simulink model "teng4_demo2_UDP_slx2py_sender_DRealTime_okclean"  (R2020a)
settings: Solver=FixedStepDiscrete  StartTime=0.0  StopTime=100  RelTol=1e-3  EnableMultiTasking=on
undefined symbols (not defined in the file or in its folder): Standard_Devices, UDP_Protocol
libraries: sldrtlib x1
Description:
  | Packet Input/Output
  | 
  | The example model "sldrtex_packetio" shows how to transfer data through
  | UDP communication protocol using binary encoding. The model sends data
  | within one computer, from one UDP port to another. You can modify the
  | model to communicate between two computers by splitting this model
  | into its send and receive parts and running the models on two computers.
  | The yellow blocks are used to send the data, the blue blocks
  | are used to receive the data. Then, please enter the host names or
  | IP addresses of the two computers into the appropriate fields
  | in the Board Setup dialog.
  | 
  | How to run this model in Normal Mode:
  | 
  | 1) Double-click the orange button to switch to Normal Mode if needed.
  | 2) Start the real-time execution using Simulation->Run.
  | 
  | How to run this model in External Mode:
  | 
  | 1) Double-click the orange button to switch to External Mode if needed.
  | 2) Start the real-time execution using Simulation->Run. The model will automatically
  |    build, connect to Simulink in External Mode and start.
settings Model: ExtModeTrigDuration=1001  Creator=The MathWorks, Inc.  LastModifiedBy=Teng
settings DataIOCC: LimitDataPoints=on  SaveFormat=Array  ReturnWorkspaceOutputs=off
settings OptimizationCC: ExpressionDepthLimit=2147483647  InitFltsAndDblsToZero=on  EfficientMapNaN2IntZero=off  LifeSpan=inf
settings DebuggingCC: UnderspecifiedInitializationDetection=Classic  MergeDetectMultiDrivingBlocksExec=none  SolverPrmCheckMsg=warning  FcnCallInpInsideContextMsg=warning  AllowSymbolicDim=off  StateNameClashWarn=warning  SFUnexpectedBacktrackingDiag=warning  SFNoUnconditionalDefaultTransitionDiag=warning  SFExecutionAtInitializationDiag=none  ArithmeticOperatorsInVariantConditions=warning
settings HardwareCC: TargetBitPerLong=64  TargetBitPerPointer=64  TargetBitPerSizeT=64  TargetBitPerPtrDiffT=64  TargetIntDivRoundTo=Zero  TargetEndianess=LittleEndian  TargetWordSize=64  TargetHWDeviceType=Intel->x86-64
settings ModelReferenceCC: PropagateSignalLabelsOutOfModel=off
settings SFSimCC: SimUseLocalCustomCode=off
settings RTWCC: Description=Simulink Desktop Real-Time  SystemTargetFile=sldrt.tlc  TemplateMakefile=sldrt.tmf  RTWUseLocalCustomCode=off  RTWCompilerOptimization=on
settings CodeAppCC: MaxIdLength=95  StateflowObjectComments=on
settings SimulinkDesktopRealTimeCC: TargetPreCompLibLocation=C:\Program Files\MATLAB\R2020a\toolbox\sldrt\lib\win64  TargetLangStandard=C89/C90 (ANSI)  SupportVariableSizeSignals=off
settings ConfigComp: CovMetricSettings=dw  CovHtmlReporting=on  CovSaveCumulativeToWorkspaceVar=on  CovSaveSingleToWorkspaceVar=on  CovShowResultsExplorer=off  CovExternalEMLEnable=off  CovSFcnEnable=off

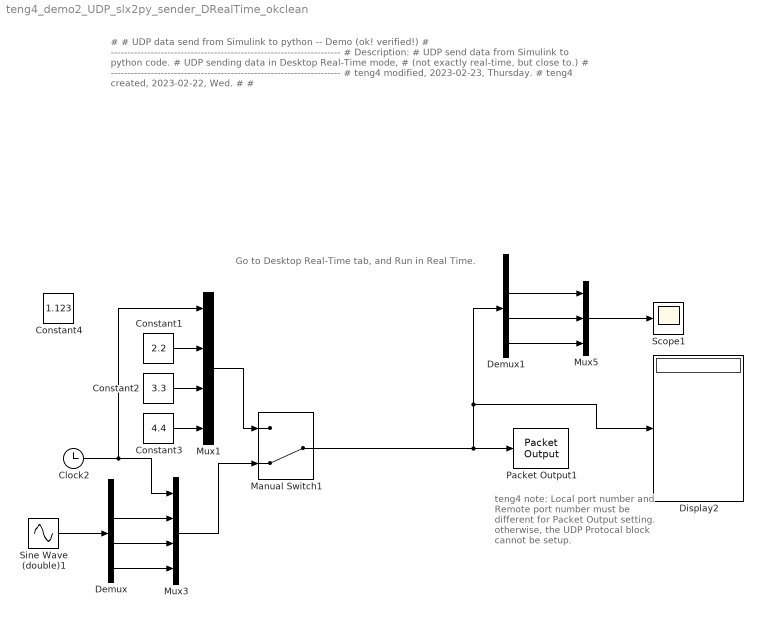
== system teng4_demo2_UDP_slx2py_sender_DRealTime_okclean ==
  note: Go to Desktop Real-Time tab,
      | and Run in Real Time.
  note: teng4 note:
      | Local port number and Remote port number must be different for Packet Output setting. otherwise, the UDP Protocal block cannot be setup.
  note: #
      | # UDP data send from Simulink to python -- Demo (ok! verified!)
      | # ---------------------------------------------------------------------
      | # Description:
      | # UDP send data from Simulink to python code.
      | # UDP sending data in Desktop Real-Time mode,
      | # (not exactly real-time, but close to.)
      | # ---------------------------------------------------------------------
      | # teng4 modified, 2023-02-23, Thursday.
      | # teng4 created, 2023-02-22, Wed.
      | #
      | #
  Clock2 : Clock
  Constant1 : Constant  Value=2.2
  Constant2 : Constant  Value=3.3
  Constant3 : Constant  Value=4.4
  Constant4 : Constant  Value=1.123
  Demux : Demux
  Demux1 : Demux
  Display2 : Display
  Manual Switch1 : ManualSwitch  CurrentSetting=0
  Mux1 : Mux
  Mux3 : Mux
  Mux5 : Mux  Inputs=3
  Packet Output1 : sldrtlib/Packet Output  SampleTime=0.1  MaxMissedTicks=Inf  ShowMissedTicks=off  YieldWhenWaiting=off  DrvName=Standard_Devices/UDP_Protocol  DrvAddress=24000  DrvOptions=[0 25000 49 57 50 46 49 54 56 46 49 46 49 48 50 0 0 0 0 0 0 0 0 0 0 0 0 0 0 0 0 0 0 0 0 0 0 0 0 0 0 0 0 0 0 0 0 0 0 0 0 0 0 0 0 0 0 0 0 0 0 0 0 0 0 0 0 0 0 0 0 0 0 0 0 0 0 0 0 0 0 0 0 0 0 0 0 0 0 0 0 0 0 0 0 0 0 0 0 0 0 0 0 0 0 0 0 0 0 0 0 0 0 0 0 0 0 0 0 0 0 0 0 0 0 0 0 0 0 0 0 0 0 0 0 0 0 0 0 0 0 0 0 0 0 0 0 0 0 0 0 0 0 0 0 0 0 0 0 0 0 0 0 0 0 0 0 0 0 0 0 0 0 0 0 0 0 0 0 0 0 0 0 0 0 0 0 0 0 0 0 0 0 0 0 0 0 0 0 0 0 0 0 0 0 0 0 0 0 0 0 0 0 0 0 0 0 0 0 0 0 0 0 0 0 0 0 0 0 0 0 0 0 0 0 0 0 0 0 0 0 0 0 0 0 0 0 0 0 0 0 0 0 0 0 0]  PacketSize=32  DataTypes={'4*double'}  ShowReady=off  ShowError=off  PacketID=1  ByteOrder=1  InitialValue=[0 0 0 0 ]  FinalValue=[0 0 0 0 ]
      settings: AttributesFormatString=UDP Protocol [24000]
  Scope1 : Scope
  Sine Wave (double)1 : Sin  Amplitude=1:4  Frequency=2  SampleTime=0
  wires:
  Sine Wave (double)1/1 -> Demux/1
  Mux1/1 -> Manual Switch1/1
  Constant3/1 -> Mux1/4
  Constant2/1 -> Mux1/3
  Constant1/1 -> Mux1/2
  Demux/2 -> Mux3/2
  Demux/3 -> Mux3/3
  Demux/4 -> Mux3/4
  Clock2/1 -> Mux1/1, Mux3/1
  Mux3/1 -> Manual Switch1/2
  Demux1/2 -> Mux5/1
  Demux1/3 -> Mux5/2
  Demux1/4 -> Mux5/3
  Mux5/1 -> Scope1/1
  Manual Switch1/1 -> Display2/1, Demux1/1, Packet Output1/1
